simulink model "FOPID"  (R2022a)
settings: Solver=VariableStepAuto  StartTime=0.0  StopTime=1  RelTol=1e-3
libraries: fod x2
settings Model: Creator=Jagadeesh  LastModifiedBy=Jagadeesh

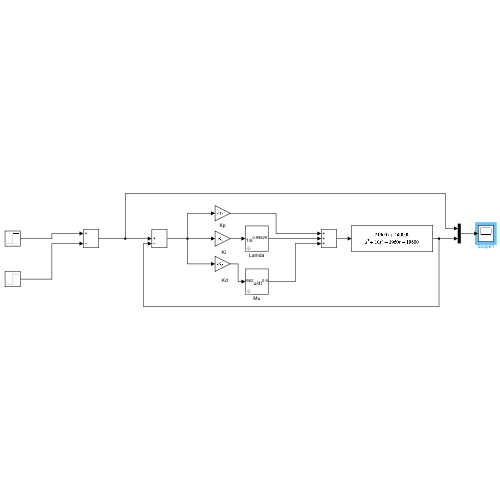
[thumbnail: Simulink's stored preview of the top-level diagram]
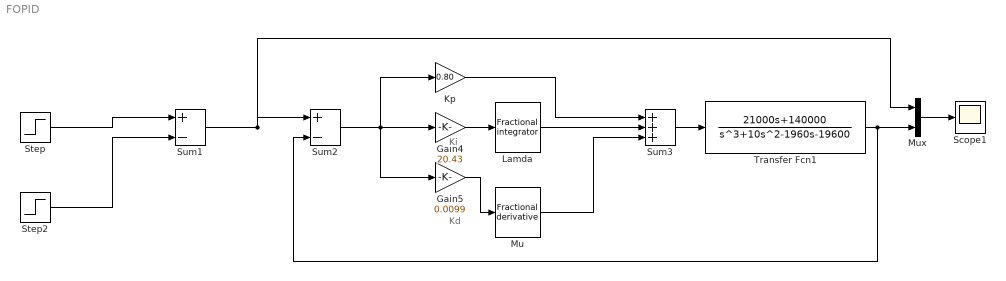
== system FOPID ==
  note: Ki
  note: Kd
  Gain4 : Gain  Gain=20.43
  Gain5 : Gain  Gain=0.0099
  Kp : Gain  Gain=0.80
  Lamda : fod/Fractional integrator  gam=0.998293  ww=[0.001; 1000]  n=5  nFod=off
      settings: SourceProductName=FOMCON Toolbox
  Mu : fod/Fractional derivative  gam=0.99562  ww=[0.001; 1000]  n=1  nFod=off
      settings: SourceProductName=FOMCON Toolbox
  Mux : Mux  Inputs=2
  Scope1 : Scope
  Step : Step  Time=0  After=0.5  SampleTime=0
  Step2 : Step  Time=0.5  After=0.3  SampleTime=0
  Sum1 : Sum  Inputs=+-
  Sum2 : Sum  Inputs=|+-
  Sum3 : Sum  Inputs=+++
  Transfer Fcn1 : TransferFcn  Numerator=[21000 140000]  Denominator=[1 10 -1960 -19600]
  wires:
  Sum3/1 -> Transfer Fcn1/1
  Lamda/1 -> Sum3/2
  Sum2/1 -> Kp/1, Gain5/1, Gain4/1
  Kp/1 -> Sum3/1
  Gain4/1 -> Lamda/1
  Gain5/1 -> Mu/1
  Mu/1 -> Sum3/3
  Transfer Fcn1/1 -> Mux/2, Sum2/2
  Mux/1 -> Scope1/1
  Step/1 -> Sum1/1
  Sum1/1 -> Sum2/1, Mux/1
  Step2/1 -> Sum1/2
